simulink model "model"  (R2022a)
settings: Solver=FixedStepAuto  StartTime=0.0  StopTime=inf  FixedStep=1  RelTol=1e-3
values from neighbouring files (symbols this model uses):
  droneCount = 3    [workspace.mat]
  map = [0 0 0 0 0 0 0 0 0 0 99 99 ... (400 elements, 20x20)]    [workspace.mat]
libraries: drone x10
settings Model: Creator=JadKHaddad  LastModifiedBy=JadKHaddad

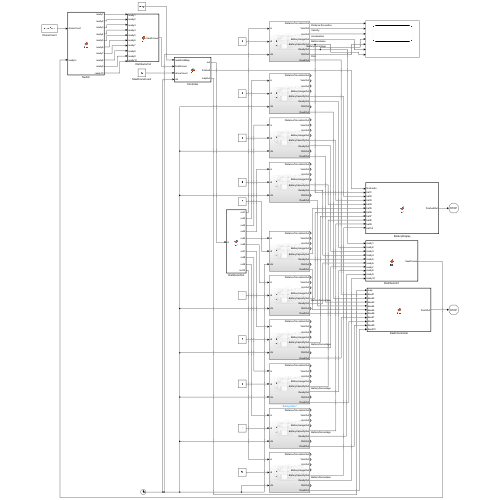
[thumbnail: Simulink's stored preview of the top-level diagram]
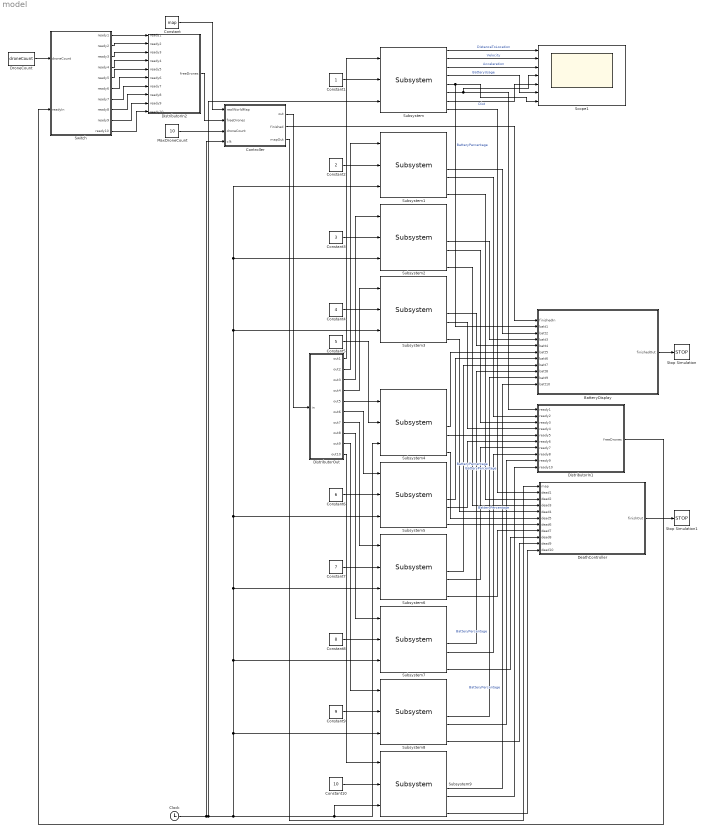
== system model ==
  BatteryDisplay : MATLAB Function  TreatAsAtomicUnit=on
  Clock : Clock
  Constant : Constant  Value=map  VectorParams1D=off
  Constant1 : Constant
  Constant10 : Constant  Value=10
  Constant2 : Constant  Value=2
  Constant3 : Constant  Value=3
  Constant4 : Constant  Value=4
  Constant5 : Constant  Value=5
  Constant6 : Constant  Value=6
  Constant7 : Constant  Value=7
  Constant8 : Constant  Value=8
  Constant9 : Constant  Value=9
  Controller : MATLAB Function  TreatAsAtomicUnit=on
  DeathController : MATLAB Function  TreatAsAtomicUnit=on
  DistributorIn1 : MATLAB Function  TreatAsAtomicUnit=on
  DistributorIn2 : MATLAB Function  TreatAsAtomicUnit=on
  DistributorOut : MATLAB Function  TreatAsAtomicUnit=on
  DroneCount : Constant  Value=droneCount
  MaxDroneCount : Constant  Value=10
  Scope1 : Scope  NumInputPorts=7
  Stop Simulation : Stop
  Stop Simulation1 : Stop
  Subsystem{,1..9} (10 alike) : drone/Subsystem  SystemSampleTime=-1  VariantActivationTime=update diagram  Latency=0  AutoFrameSizeCalculation=off
  Switch : MATLAB Function  TreatAsAtomicUnit=on
  wires:
  Subsystem9/5 -> BatteryDisplay/11(batt10)  "BatteryPercentage"
  Subsystem3/8 -> DeathController/5(dead4)
  Subsystem9/6 -> DistributorIn1/10(ready10)
  Subsystem8/5 -> BatteryDisplay/10(batt9)  "BatteryPercentage"
  Constant7/1 -> Subsystem6/2
  Subsystem5/6 -> DistributorIn1/6(ready6)
  Subsystem7/5 -> BatteryDisplay/9(batt8)  "BatteryPercentage"
  Switch/8(ready8) -> DistributorIn2/8(ready8)
  Subsystem4/6 -> DistributorIn1/5(ready5)
  Subsystem6/5 -> BatteryDisplay/8(batt7)  "BatteryPercentage"
  Subsystem5/5 -> BatteryDisplay/7(batt6)  "BatteryPercentage"
  Constant10/1 -> Subsystem9/2
  Subsystem7/6 -> DistributorIn1/8(ready8)
  Constant4/1 -> Subsystem3/2
  Subsystem2/6 -> DistributorIn1/3(ready3)
  Subsystem8/6 -> DistributorIn1/9(ready9)
  Subsystem6/6 -> DistributorIn1/7(ready7)
  Subsystem9/8 -> DeathController/11(dead10)
  Subsystem4/8 -> DeathController/6(dead5)
  Subsystem8/8 -> DeathController/10(dead9)
  Switch/10(ready10) -> DistributorIn2/10(ready10)
  Subsystem7/8 -> DeathController/9(dead8)
  Subsystem6/8 -> DeathController/8(dead7)
  Subsystem5/8 -> DeathController/7(dead6)
  MaxDroneCount/1 -> Controller/3(droneCount)
  DistributorOut/10(out10) -> Subsystem9/1
  DistributorOut/9(out9) -> Subsystem8/1
  DistributorOut/8(out8) -> Subsystem7/1
  Subsystem/3 -> Scope1/3  "Acceleration"
  DistributorOut/7(out7) -> Subsystem6/1
  DistributorOut/6(out6) -> Subsystem5/1
  Constant6/1 -> Subsystem5/2
  Constant8/1 -> Subsystem7/2
  Constant9/1 -> Subsystem8/2
  Switch/9(ready9) -> DistributorIn2/9(ready9)
  Switch/7(ready7) -> DistributorIn2/7(ready7)
  Switch/6(ready6) -> DistributorIn2/6(ready6)
  DeathController/1(finishOut) -> Stop Simulation1/1
  Subsystem3/6 -> DistributorIn1/4(ready4)
  Constant2/1 -> Subsystem1/2
  Subsystem2/8 -> DeathController/4(dead3)
  Subsystem1/8 -> DeathController/3(dead2)
  Constant/1 -> Controller/1(realWorldMap)
  Switch/2(ready2) -> DistributorIn2/2(ready2)
  Subsystem4/5 -> BatteryDisplay/6(batt5)
  Subsystem/1 -> Scope1/1  "DistanceToLocation"
  Subsystem3/5 -> BatteryDisplay/5(batt4)
  Constant5/1 -> Subsystem4/2
  DistributorOut/2(out2) -> Subsystem1/1
  DistributorOut/4(out4) -> Subsystem3/1
  DistributorIn2/1(freeDrones) -> Controller/2(freeDrones)
  Controller/1(out) -> DistributorOut/1(in)
  Subsystem/4 -> Scope1/6  "BatteryUsage"
  Subsystem/8 -> DeathController/2(dead1)
  Constant3/1 -> Subsystem2/2
  BatteryDisplay/1(finishedOut) -> Stop Simulation/1
  Constant1/1 -> Subsystem/2
  DistributorIn1/1(freeDrones) -> Switch/2(readyIn)
  Subsystem/2 -> Scope1/2  "Velocity"
  Controller/3(mapOut) -> DeathController/1(map)
  Controller/2(finished) -> BatteryDisplay/1(finishedIn)
  Subsystem/7 -> Scope1/5  "Dist"
  Subsystem1/6 -> DistributorIn1/2(ready2)
  DistributorOut/3(out3) -> Subsystem2/1
  DroneCount/1 -> Switch/1(droneCount)
  DistributorOut/1(out1) -> Subsystem/1
  Switch/3(ready3) -> DistributorIn2/3(ready3)
  Switch/1(ready1) -> DistributorIn2/1(ready1)
  Switch/4(ready4) -> DistributorIn2/4(ready4)
  Subsystem2/5 -> BatteryDisplay/4(batt3)
  DistributorOut/5(out5) -> Subsystem4/1
  Subsystem1/5 -> BatteryDisplay/3(batt2)
  Switch/5(ready5) -> DistributorIn2/5(ready5)
  Subsystem/5 -> Scope1/7, BatteryDisplay/2(batt1)  "BatteryPercentage"
  Subsystem/6 -> Scope1/4, DistributorIn1/1(ready1)
  Clock/1 -> Subsystem4/3, Subsystem9/3, Subsystem1/3, Subsystem2/3, Subsystem3/3, Subsystem5/3, Subsystem6/3, Subsystem7/3, Subsystem8/3, Subsystem/3, Controller/4(clk)

== matlab function model/DistributorIn1 ==
  data: ready1 input; freeDrones output; ready2 input; ready3 input; ready4 input; ready5 input; ready6 input; ready7 input; ready8 input; ready9 input; ready10 input
function freeDrones = fcn(ready1, ready2, ready3, ready4, ready5, ready6, ready7, ready8, ready9, ready10)
    freeDrones = [ready1 ready2 ready3 ready4 ready5 ready6 ready7 ready8 ready9 ready10];
end

== matlab function model/Controller ==
  settings: updateMethod=DISCRETE
  data: realWorldMap input; out output; finished output; freeDrones input; droneCount input; mapOut output; clk input
function [out, finished, mapOut] = fcn(realWorldMap, freeDrones, droneCount, clk)
    persistent index
    persistent indexLimit
    persistent path
    persistent lastXY
    persistent workingDronesCount
    persistent cameBackDronesCount
    persistent map
    persistent workingDrones
    persistent inTermMode
    
    if isempty(inTermMode)
        inTermMode = 0;
    end
    if isempty(workingDrones)
        workingDrones = zeros(droneCount);
    end
    if isempty(workingDronesCount)
        workingDronesCount = 0;
    end
    if isempty(cameBackDronesCount)
        cameBackDronesCount = 0;
    end
    if isempty(index)
        index = 1;
    end
    if isempty(indexLimit)
        indexLimit = 2;
    end
    if isempty(path)
        path = ones(length(realWorldMap)*length(realWorldMap),2);
    end
    if isempty(lastXY)
        lastXY = ones(droneCount, 2);
        lastXY = -1 * lastXY;
    end
    if isempty(map)
        map = zeros(length(realWorldMap), length(realWorldMap));
    end

    function indexDist = getIndexAndDistOfAFreeDrone(dest)
        DIndex = -1;
        minDist = -1;
        i = 1;
        while(i <= droneCount)
            if(freeDrones(i) == 1)
                source = lastXY(i,:);
                if source(1) == -2
                    i = i + 1;
                    continue
                end
                if(source(1) == -1)
                    source(1) = 1;
                end
                if(source(2) == -1)
                    source(2) = 1;
                end
                dist = minDistanceSimulink(map, source(1), source(2), dest(1), dest(2));
                if(minDist == -1 && dist ~= -1) || (minDist ~= -1 && dist ~= -1 && dist < minDist)
                    minDist = dist;
                    DIndex = i;
                end
            end
            i = i + 1;
        end
        indexDist = [DIndex minDist];
    end

    finished = 0;
    mapOut = map;

    %out = [xy(1) xy(2) dist vld];
    out = ones(10, 4);
    i = 1;
    while (i <= droneCount)
       out(i,:) = [1 1 -1 0];
       i = i + 1;
    end

    %sink
    if cameBackDronesCount >= droneCount
        finished = 1;
        fprintf("[%d]: All drones came back. Terminating...\n\nMap:\n", int32(clk));
        disp(map);
        return
    end
    i = 1;
    while i <= droneCount
        x = lastXY(i, 1);
        y = lastXY(i, 2);
        droneIsFree = freeDrones(1, i);
        if droneIsFree == 1 && x == -2
            cameBackDronesCount = cameBackDronesCount + 1;
            fprintf("[%d]: Drone [%d] came back\n", int32(clk), int8(i));
            lastXY(i,:) = [-3 -3];
            i = i + 1;
            continue
        end
        if droneIsFree == 1 && x ~= -1 && x ~= -2 && x ~= -3 && workingDrones(i) == 1
            %update path
            fprintf("[%d]: Drone [%d] is now ready\n", int32(clk), int8(i));
            workingDrones(i) = 0;
            workingDronesCount = workingDronesCount - 1;
            map(x,y) = 3;
            if realWorldMap(x,y) == 0
                if x + 1 <= length(realWorldMap) && map(x + 1, y) == 0
                    if realWorldMap(x + 1, y) == 0
                        newRow = [x+1 y];
                        map(x+1,y) = -1;
                        path(indexLimit,:) = newRow;
                        indexLimit = indexLimit + 1;
                    else
                        map(x+1,y) = 99;
                    end
                end
                
                if y + 1 <= length(realWorldMap) && map(x, y + 1) == 0
                    if realWorldMap(x, y + 1) == 0
                        newRow = [x y+1];
                        map(x,y+1) = -1;
                        path(indexLimit,:) = newRow;
                        indexLimit = indexLimit + 1;
                    else
                        map(x, y + 1) = 99;
                    end
                end
                
                if x - 1 >= 1 && map(x - 1, y) == 0 
                    if realWorldMap(x - 1, y) == 0 
                        newRow = [x-1 y];
                        map(x-1,y) = -1;
                        path(indexLimit,:) = newRow;
                        indexLimit = indexLimit + 1;
                    else
                        map(x - 1, y) = 99;
                    end
                end
                
                if y - 1 >= 1 && map(x, y-1) == 0
                    if realWorldMap(x, y-1) == 0
                        newRow = [x y-1];
                        map(x,y-1) = -1;
                        path(indexLimit,:) = newRow;
                        indexLimit = indexLimit + 1;
                    else
                        map(x, y-1) = 99;
                    end
                end
            end
            j = index;
            fprintf("[%d]: Next free positions: ", int32(clk));
            while j < indexLimit
                fprintf("(%d, %d) ", int8(path(j,1)), int8(path(j,2)));
                j = j + 1;
            end
            fprintf("\n");
        end
        i = i + 1;
    end

    if index >= indexLimit
        if workingDronesCount == 0
            if inTermMode == 0
                fprintf("[%d]: Entering termination mode\n", int32(clk));
                inTermMode = 1;
            end
            droneIndex = 1;
            while droneIndex <= droneCount
                droneLocation = lastXY(droneIndex,:);
                if droneLocation(1) == -1
                    fprintf("[%d]: Drone [%d] is already at start location\n", int32(clk), int8(droneIndex));
                    lastXY(droneIndex, :) = [-3 -3];
                    cameBackDronesCount = cameBackDronesCount + 1;
                    droneIndex = droneIndex + 1;
                    continue
                end
                if droneLocation(1) == -3 || droneLocation(1) == -2
                    droneIndex = droneIndex + 1;
                    continue
                end
                droneIsFree = freeDrones(1, droneIndex);
                if droneIsFree == 1
                    dist = minDistanceSimulink(map, droneLocation(1), droneLocation(2), 1, 1);
                    out(droneIndex,1) = -2;
                    out(droneIndex,2) = -2;
                    out(droneIndex,3) = dist;
                    out(droneIndex,4) = 1;
                    fprintf("[%d]: Calling drone [%d] back from(%d, %d) with distance [%d]\n", int32(clk), int8(droneIndex), int8(lastXY(droneIndex,1)), int8(lastXY(droneIndex,2)), int8(dist));
    
                    map(droneLocation(1), droneLocation(2)) = 1;
                    lastXY(droneIndex,:) = [-2 -2];
                end
                droneIndex = droneIndex + 1;
            end
        end

    else
        dest = path(index,:);
        indexDist = getIndexAndDistOfAFreeDrone(dest);
        droneIndex = indexDist(1);
        dist = indexDist(2);
        if droneIndex > -1 && dist > -1
            out(droneIndex,1) = dest(1);
            out(droneIndex,2) = dest(2);
            out(droneIndex,3) = dist;
            out(droneIndex,4) = 1;
            fprintf("[%d]: Sending drone [%d] from (%d, %d) to (%d, %d) with distance [%d]\n", int32(clk), int8(droneIndex), int8(lastXY(droneIndex,1)), int8(lastXY(droneIndex,2)), int8(dest(1)), int8(dest(2)), int8(dist));
            workingDronesCount = workingDronesCount + 1;
            workingDrones(droneIndex) = 1;
            if lastXY(droneIndex,1) ~= -1
                if map(lastXY(droneIndex,1), lastXY(droneIndex,2)) == 3
                    map(lastXY(droneIndex,1), lastXY(droneIndex,2)) = 1;
                end
            end
            map(dest(1),dest(2)) = 2;
            lastXY(droneIndex,:) = dest;
            index = index + 1;
        end
    end
end

== matlab function model/DistributorOut ==
  data: in input; out1 output; out2 output; out3 output; out4 output; out5 output; out6 output; out7 output; out8 output; out9 output; out10 output
function [out1, out2, out3, out4, out5, out6, out7, out8, out9, out10] = fcn(in)
    out1 = [1 1 -1 0];
    out2 = [1 1 -1 0];    
    out3 = [1 1 -1 0];
    out4 = [1 1 -1 0];    
    out5 = [1 1 -1 0];
    out6 = [1 1 -1 0];
    out7 = [1 1 -1 0];    
    out8 = [1 1 -1 0];
    out9 = [1 1 -1 0];    
    out10 = [1 1 -1 0];
    
    out1 = in(1,:);
    out2 = in(2,:);
    out3 = in(3,:);
    out4 = in(4,:);
    out5 = in(5,:);
    out6 = in(6,:);
    out7 = in(7,:);
    out8 = in(8,:);
    out9 = in(9,:);
    out10 = in(10,:);
end

== matlab function model/DistributorIn2 ==
  data: ready1 input; freeDrones output; ready2 input; ready3 input; ready4 input; ready5 input; ready6 input; ready7 input; ready8 input; ready9 input; ready10 input
function freeDrones = fcn(ready1, ready2, ready3, ready4, ready5, ready6, ready7, ready8, ready9, ready10)
    freeDrones = [ready1 ready2 ready3 ready4 ready5 ready6 ready7 ready8 ready9 ready10];
end

== matlab function model/BatteryDisplay ==
  data: finishedIn input; finishedOut output; batt1 input; batt2 input; batt3 input; batt4 input; batt5 input; batt6 input; batt7 input; batt8 input; batt9 input; batt10 input
function finishedOut = fcn(finishedIn, batt1, batt2, batt3, batt4, batt5, batt6, batt7, batt8, batt9, batt10)

finishedOut = finishedIn;

if finishedIn == 1
    fprintf("\n\n");
    fprintf("Drone [1] battery capacity: [%f%%]\n", batt1*100);
    fprintf("Drone [2] battery capacity: [%f%%]\n", batt2*100);
    fprintf("Drone [3] battery capacity: [%f%%]\n", batt3*100);
    fprintf("Drone [4] battery capacity: [%f%%]\n", batt4*100);
    fprintf("Drone [5] battery capacity: [%f%%]\n", batt5*100);
    fprintf("Drone [6] battery capacity: [%f%%]\n", batt6*100);
    fprintf("Drone [7] battery capacity: [%f%%]\n", batt7*100);
    fprintf("Drone [8] battery capacity: [%f%%]\n", batt8*100);
    fprintf("Drone [9] battery capacity: [%f%%]\n", batt9*100);
    fprintf("Drone [10] battery capacity: [%f%%]\n", batt10*100);
end

== matlab function model/DeathController ==
  data: map input; finishOut output; dead1 input; dead2 input; dead3 input; dead4 input; dead5 input; dead6 input; dead7 input; dead8 input; dead9 input; dead10 input
function finishOut = fcn(map, dead1, dead2, dead3, dead4, dead5, dead6, dead7, dead8, dead9, dead10)
allDead = 0;

if dead1 == 1 && dead2 == 1 && dead3 == 1 && dead4 == 1 && dead5 == 1 && dead6 == 1 && dead7 == 1 && dead8 == 1 && dead9 == 1 && dead10 == 1
    allDead = 1;
end

if allDead == 1
    fprintf("All drones died. Terminating...\n\nMap:\n");
    disp(map);
end

finishOut = allDead;

== matlab function model/Switch ==
  data: droneCount input; ready1 output; readyIn input; ready2 output; ready3 output; ready4 output; ready5 output; ready6 output; ready7 output; ready8 output; ready9 output; ready10 output
function [ready1, ready2, ready3, ready4, ready5, ready6, ready7, ready8, ready9, ready10] = fcn(droneCount, readyIn)

    out = zeros(10);
    i = 1;
    while i <= droneCount
        out(i) = readyIn(i);
        i = i +1;
    end
    
    ready1 = out(1);
    ready2 = out(2);
    ready3 = out(3);
    ready4 = out(4);
    ready5 = out(5);
    ready6 = out(6);
    ready7 = out(7);
    ready8 = out(8);
    ready9 = out(9);
    ready10 = out(10);
    
end
